simulink model "Horizontal_Rolling_Tongji_Model"  (R2021b)
settings: Solver=ode15s  StartTime=0.0  StopTime=50  FixedStep=1e-4  MaxStep=1e-5  RelTol=1e-5
values from neighbouring files (symbols this model uses):
  J_1 = m_1*r_1^2/2    (= 0.1)    [Horizontal_Rolling_Tongji.m]
  J_2 = m_2*r_2^2/2    (= 2.5)    [Horizontal_Rolling_Tongji.m]
  mu_d = 0.5    [Horizontal_Rolling_Tongji.m]
  mu_r = mu_s*10^-2    (= 0.0065)    [Horizontal_Rolling_Tongji.m]
  mu_s = 0.65    [Horizontal_Rolling_Tongji.m]
  N = 50    [Horizontal_Rolling_Tongji.m]
  r_1 = 0.2    [Horizontal_Rolling_Tongji.m]
  r_2 = 0.5    [Horizontal_Rolling_Tongji.m]
libraries: simulink x4
settings Model: Creator=Gioele  LastModifiedBy=gioele
settings SolverCC: AlgebraicLoopSolver=LineSearch
settings DebuggingCC: SFMachineParentedDataDiag=warning

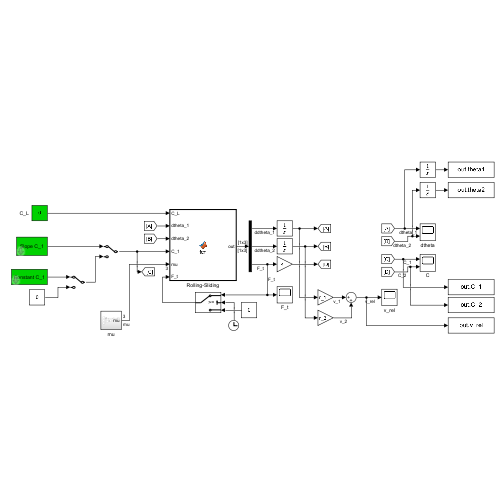
[thumbnail: Simulink's stored preview of the top-level diagram]
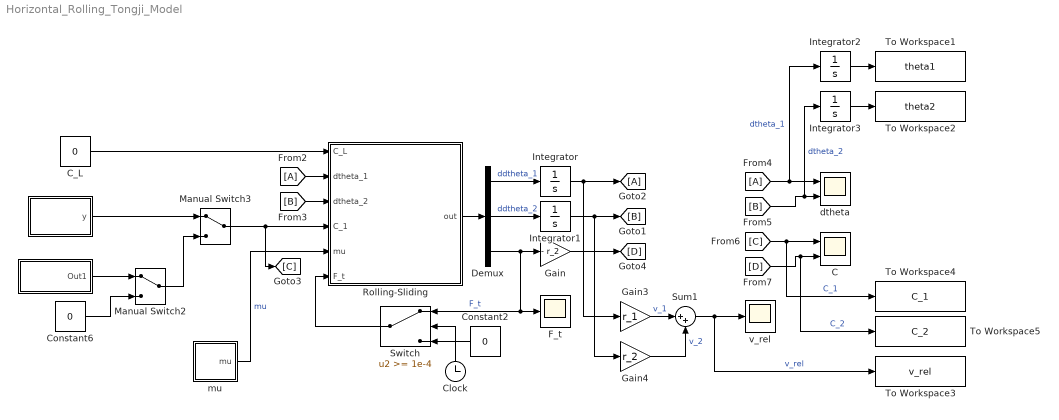
== system Horizontal_Rolling_Tongji_Model ==
  " " : Subsystem  mask{C_1_slope_gain=1.0}
      mask prompts: C_1_slope_gain "Slope C_1 gain"
      mask Display: disp('Slope C_1')
  "  " : Subsystem  mask{C_1_constant=1}
      mask prompts: C_1_constant "Constant C_1"
      mask Display: disp('Constant C_1')
  C : Scope  NumInputPorts=2
  C_L : Constant  Value=0
  Clock : Clock
  Constant2 : Constant  Value=0
  Constant6 : Constant  Value=0
  Demux : Demux  Outputs=3
  F_t : Scope
  Gain : Gain  Gain=- r_2
  Gain3 : Gain  Gain=r_1
  Gain4 : Gain  Gain=r_2
  Integrator{,1..3} (4 alike) : Integrator
  Manual Switch2 : ManualSwitch
  Manual Switch3 : ManualSwitch
  Rolling-Sliding : MATLAB Function  TreatAsAtomicUnit=on
  Sum1 : Sum  Inputs=|++
  Switch : Switch  Threshold=1e-4
  To Workspace1 : ToWorkspace  VariableName=theta1  SampleTime=1e-2
  To Workspace2 : ToWorkspace  VariableName=theta2  SampleTime=1e-2
  To Workspace3 : ToWorkspace  VariableName=v_rel  SampleTime=1e-2
  To Workspace4 : ToWorkspace  VariableName=C_1  SampleTime=1e-2
  To Workspace5 : ToWorkspace  VariableName=C_2  SampleTime=1e-2
  dtheta : Scope  NumInputPorts=2
  mu : Subsystem
  v_rel : Scope
  wires:
  Demux/1 -> Integrator/1  "ddtheta_1"
  Demux/2 -> Integrator1/1  "ddtheta_2"
  Integrator/1 -> [A], Gain3/1
  Integrator1/1 -> [B], Gain4/1
  Demux/3 -> F_t/1, Switch/1, Gain/1  "F_t"
  Gain/1 -> [D]
  Gain3/1 -> Sum1/1  "v_1"
  Gain4/1 -> Sum1/2  "v_2"
  Sum1/1 -> To Workspace3/1, v_rel/1  "v_rel"
  Rolling-Sliding/1(out) -> Demux/1
  [B] -> Rolling-Sliding/3(dtheta_2)
  [A] -> Rolling-Sliding/2(dtheta_1)
  [A] -> Integrator2/1, dtheta/1  "dtheta_1"
  [B] -> Integrator3/1, dtheta/2  "dtheta_2"
  [D] -> To Workspace5/1, C/2  "C_2"
  [C] -> To Workspace4/1, C/1  "C_1"
  Manual Switch3/1 -> [C], Rolling-Sliding/4(C_1)
  mu/1(mu) -> Rolling-Sliding/5(mu)  "mu"
  Switch/1 -> Rolling-Sliding/6(F_t)
  Constant2/1 -> Switch/3
  Clock/1 -> Switch/2
  " "/1(y) -> Manual Switch3/1
  Constant6/1 -> Manual Switch2/2
  Manual Switch2/1 -> Manual Switch3/2
  "  "/1(Out1) -> Manual Switch2/1
  C_L/1 -> Rolling-Sliding/1(C_L)
  Integrator2/1 -> To Workspace1/1
  Integrator3/1 -> To Workspace2/1

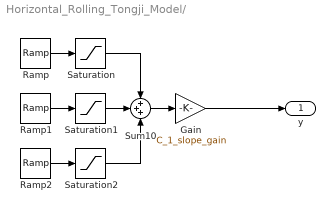
== system Horizontal_Rolling_Tongji_Model/  ==
  Gain : Gain  Gain=C_1_slope_gain
  Ramp : simulink/Sources/Ramp  slope=1  start=5  InitialOutput=0
  Ramp1 : simulink/Sources/Ramp  slope=1  start=15  InitialOutput=0
  Ramp2 : simulink/Sources/Ramp  slope=-1  start=25  InitialOutput=0
  Saturation : Saturate  UpperLimit=5  LowerLimit=0
  Saturation1 : Saturate  UpperLimit=5  LowerLimit=0
  Saturation2 : Saturate  UpperLimit=0  LowerLimit=-10
  Sum10 : Sum  Inputs=+++
  y : Outport
  wires:
  Saturation1/1 -> Sum10/2
  Sum10/1 -> Gain/1
  Ramp1/1 -> Saturation1/1
  Saturation/1 -> Sum10/1
  Ramp2/1 -> Saturation2/1
  Ramp/1 -> Saturation/1
  Gain/1 -> y/1
  Saturation2/1 -> Sum10/3

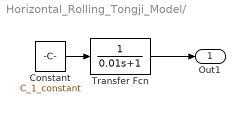
== system Horizontal_Rolling_Tongji_Model/   ==
  Constant : Constant  Value=C_1_constant
  Transfer Fcn : TransferFcn  Denominator=[0.01 1]
  Out1 : Outport
  wires:
  Constant/1 -> Transfer Fcn/1
  Transfer Fcn/1 -> Out1/1

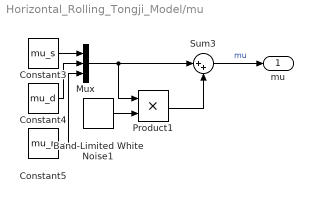
== system Horizontal_Rolling_Tongji_Model/mu ==
  Band-Limited White Noise1 : simulink/Sources/Band-Limited White Noise  Cov=[0.000001]  Ts=0.1  seed=[23341]
  Constant3 : Constant  Value=mu_s
  Constant4 : Constant  Value=mu_d
  Constant5 : Constant  Value=mu_r
  Mux : Mux  Inputs=3
  Product1 : Product
  Sum3 : Sum  Inputs=|++
  mu : Outport
  wires:
  Sum3/1 -> mu/1  "mu"
  Constant5/1 -> Mux/3
  Band-Limited White Noise1/1 -> Product1/2
  Constant4/1 -> Mux/2
  Product1/1 -> Sum3/2
  Constant3/1 -> Mux/1
  Mux/1 -> Sum3/1, Product1/1

== matlab function Horizontal_Rolling_Tongji_Model/Rolling-Sliding ==
  data: C_L input; dtheta_1 input; dtheta_2 input; C_1 input; r_1 parameter; r_2 parameter; J_1 parameter; J_2 parameter; N parameter; mu input; F_t input; out output
function out = fcn(C_L,dtheta_1,dtheta_2,C_1,r_1,r_2,J_1,J_2,N,mu,F_t)
% function out = fcn(dtheta_1,dtheta_2,ddtheta_1,ddtheta_2,tau,r_1,r_2,J_1,J_2,N, mu)

mu_s_n = mu(1);
mu_d_n = mu(2);
mu_r_n = mu(3);

if abs(dtheta_1) > 0.001
    C_rf1 = - sign(dtheta_1)*mu_r_n*N;
else
    if abs(C_1) < mu_r_n*N
        C_rf1 = - C_1;
    else
        C_rf1 = - sign(dtheta_1)*mu_r_n*N;
    end
end
if abs(dtheta_2) > 0.001
    C_rf2 = - sign(dtheta_2)*mu_r_n*N;
else
%     if abs(((tau*J_2*r_1 + C_rf1*J_2*r_1 + (((tau*J_2*r_1 + C_rf1*J_2*r_1)/(J_2*r_1^2 + J_1*r_2^2))*r_2)*J_1*r_2)/(J_2*r_1^2 + J_1*r_2^2))*r_2) < mu_r_n*N
%         C_rf2 = ((tau*J_2*r_1 + C_rf1*J_2*r_1)/(J_2*r_1^2 + J_1*r_2^2))*r_2;
    if abs(- F_t*r_2) < mu_r_n*N
        C_rf2 = - (- F_t*r_2);
    else
        C_rf2 = - sign(dtheta_2)*mu_r_n*N;
    end
end

if (-0.001 < dtheta_1*r_1 + dtheta_2*r_2) && (dtheta_1*r_1 + dtheta_2*r_2 < 0.001)
    % Condition should be (dtheta_1*r_1 + dtheta_2*r_2 == 0) but need
    % tolerance for simulation reasons
    F_t = (C_1*J_2*r_1 + C_rf1*J_2*r_1 + C_rf2*J_1*r_2 + C_L*J_1*r_2)/(J_2*r_1^2 + J_1*r_2^2);
    % Pure rolling case
    if (abs(F_t) > mu_s_n*N)
        F_t = sign(dtheta_1*r_1 + dtheta_2*r_2)*mu_d_n*N;
        % Transition from Rolling to Rolling with sliding
    end
else
    F_t = sign(dtheta_1*r_1 + dtheta_2*r_2)*mu_d_n*N;
    % Rolling with sliding case
end

ddtheta_1 = (C_1 + C_rf1 - F_t*r_1)/(J_1);
ddtheta_2 = (- F_t*r_2 + C_rf2 + C_L)/(J_2);

out = [ddtheta_1,ddtheta_2,F_t];
